simulink model "enu"  (R2016a)
settings: Solver=FixedStepDiscrete  StartTime=0.0  StopTime=10.0  RelTol=1e-3
undefined symbols (not defined in the file or in its folder): number
libraries: simulink x2
settings Model: Creator=hp  LastModifiedBy=hp
settings OptimizationCC: DefaultParameterBehavior=Inlined  OptimizeModelRefInitCode=on  LifeSpan=1
settings DebuggingCC: UnderspecifiedInitializationDetection=Classic  MergeDetectMultiDrivingBlocksExec=none
settings ModelReferenceCC: PropagateSignalLabelsOutOfModel=off
settings RTWCC: SystemTargetFile=ert.tlc  GenCodeOnly=on  TemplateMakefile=ert_default_tmf  GenerateReport=on  IncludeHyperlinkInReport=on  LaunchReport=on  GenerateTraceInfo=on  GenerateTraceReport=on  GenerateTraceReportSl=on  GenerateTraceReportSf=on  GenerateTraceReportEml=on
settings CodeAppCC: ForceParamTrailComments=on  IgnoreCustomStorageClasses=off  OperatorAnnotations=on  SimulinkDataObjDesc=on  SFDataObjDesc=on  MATLABFcnDesc=on  InsertBlockDesc=on  MATLABSourceComments=on
settings ERTTargetCC: GenerateSampleERTMain=on  InlinedParameterPlacement=NonHierarchical  ERTCustomFileTemplate=example_file_process.tlc

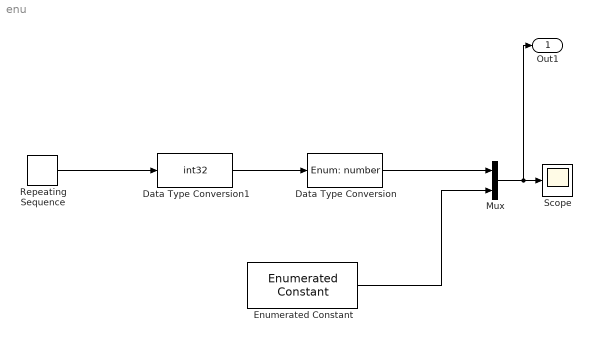
== system enu ==
  Data Type Conversion : DataTypeConversion  OutDataTypeStr=Enum: number
  Data Type Conversion1 : DataTypeConversion  OutDataTypeStr=int32
  Enumerated Constant : simulink/Sources/Enumerated Constant  OutDataTypeStr=Enum: number  Value=number.two  SampleTime=inf
  Mux : Mux  Inputs=2
  Repeating Sequence : simulink/Sources/Repeating Sequence  rep_seq_t=[0 1 2 3 4 5]  rep_seq_y=[0 1 2 1 0 3]
  Scope : Scope
  Out1 : Outport
  wires:
  Mux/1 -> Out1/1, Scope/1
  Data Type Conversion/1 -> Mux/1
  Data Type Conversion1/1 -> Data Type Conversion/1
  Enumerated Constant/1 -> Mux/2
  Repeating Sequence/1 -> Data Type Conversion1/1
